simulink subsystem "cvrs_frank_starling"  (R2020b)
settings: Solver=VariableStepAuto  StartTime=0.0  StopTime=10.0  RelTol=1e-3
settings Model: Creator=RH  LastModifiedBy=Marco

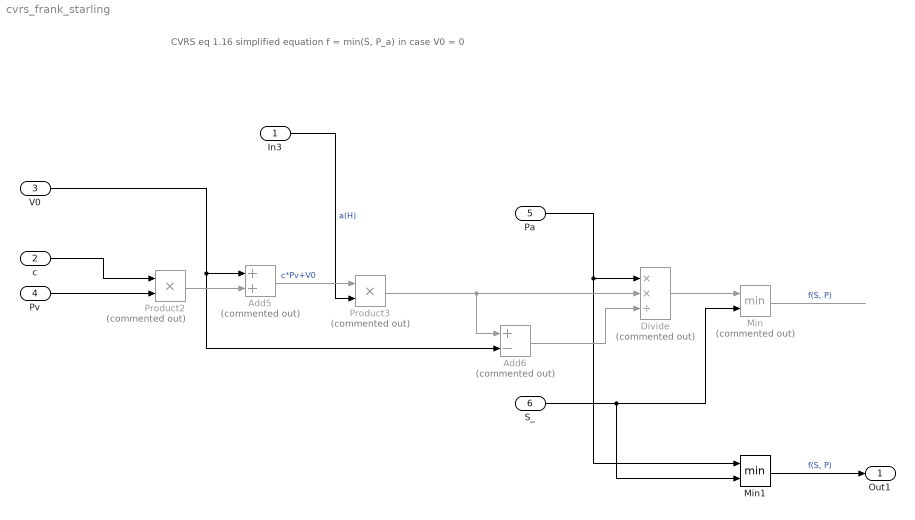
== system cvrs_frank_starling ==
  note: CVRS eq 1.16
      | simplified equation f = min(S, P_a) in case V0 = 0
  In3 : Inport
  c : Inport  Port=2
  V0 : Inport  Port=3
  Pv : Inport  Port=4
  Pa : Inport  Port=5
  S_ : Inport  Port=6
  Add5 : Sum  Commented=on
  Add6 : Sum  Commented=on  Inputs=+-
  Divide : Product  Commented=on  Inputs=**/
  Min : MinMax  Commented=on  Inputs=2
  Min1 : MinMax  Inputs=2
  Product2 : Product  Commented=on
  Product3 : Product  Commented=on
  Out1 : Outport
  wires:
  In3/1 -> Product3/2  "a(H)"
  Pv/1 -> Product2/2
  Min/1 -> ?  "f(S, P)"
  Pa/1 -> Divide/1, Min1/1
  c/1 -> Product2/1
  Add6/1 -> Divide/3
  S_/1 -> Min/2, Min1/2
  Divide/1 -> Min/1
  V0/1 -> Add6/2, Add5/1
  Product3/1 -> Add6/1, Divide/2
  Product2/1 -> Add5/2
  Add5/1 -> Product3/1  "c*Pv+V0"
  Min1/1 -> Out1/1  "f(S, P)"
